simulink model "PMSM_FOC_INVERTER_COMPARISON"  (R2023b)
settings: Solver=VariableStepAuto  StartTime=0.0  StopTime=1  RelTol=1e-3
InitFcn:
  | Ld = 1.7e-3;
  | Lq = 3.2e-3;
  | Rs = 0.02;
  | Lambda_m = 0.2205;
  | J = 0.0027;
  | P = 4;
  | B = 0.001;
  | Vdc = 500;
libraries: slpidlib x9, spsControlledVoltageSourceLib x3, spsGroundLib x3, spsVoltageMeasurementLib x3, spsDCVoltageSourceLib x1, spsPermanentMagnetSynchronousMachineLib x1, spsUniversalBridgeLib x1, sps_lib x1, spsTriangleGeneratorLib x1
(part 2 of 2)

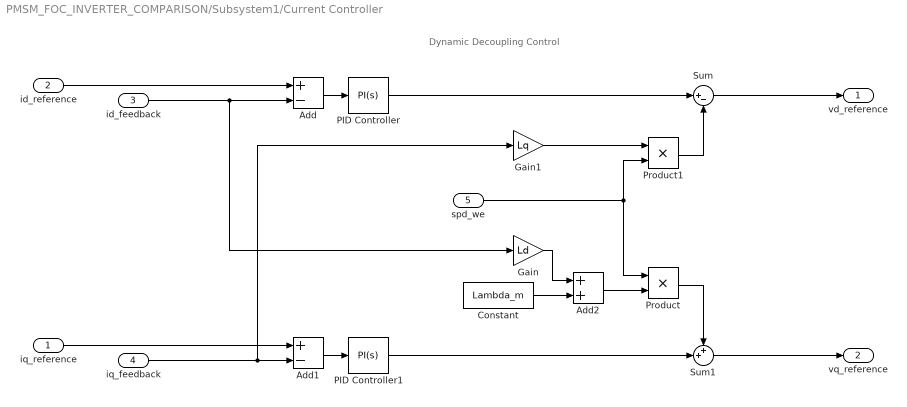
== system PMSM_FOC_INVERTER_COMPARISON/Subsystem1/Current Controller ==
  note: Dynamic Decoupling Control
  iq_reference : Inport  SampleTime=1e-4
  id_reference : Inport  Port=2  SampleTime=1e-4
  id_feedback : Inport  Port=3  SampleTime=1e-4
  iq_feedback : Inport  Port=4  SampleTime=1e-4
  spd_we : Inport  Port=5  SampleTime=1e-4
  Add : Sum  Inputs=+-
  Add1 : Sum  Inputs=+-
  Add2 : Sum
  Constant : Constant  Value=Lambda_m  SampleTime=1e-4
  Gain : Gain  Gain=Ld
  Gain1 : Gain  Gain=Lq
  PID Controller : slpidlib/PID Controller  Controller=PI  Form=Parallel  TimeDomain=Continuous-time  UseExternalTs=off  SampleTime=-1  IntegratorMethod=Forward Euler  FilterMethod=Forward Euler  ControllerParametersSource=internal  P=7.74  I=26.84  UseKiTs=off  D=0  N=100  UseFilter=on  TunerSelectOption=Transfer Function Based (PID Tuner App)  InitialConditionSource=internal  InitialConditionForIntegrator=0  InitialConditionForFilter=0  DifferentiatorICPrevScaledInput=0  ExternalReset=none  TrackingMode=off  Kt=1  LimitOutput=off  SatLimitsSource=internal  UpperSaturationLimit=inf  LowerSaturationLimit=-inf  LinearizeAsGain=on  AntiWindupMode=none  Kb=1  LimitIntegrator=off  UpperIntegratorSaturationLimit=inf  LowerIntegratorSaturationLimit=-inf  POutMin=[]  POutMax=[]  IOutMin=[]  IOutMax=[]  DOutMin=[]  DOutMax=[]  NOutMin=[]  NOutMax=[]  SumOutMin=[]  SumOutMax=[]  SaturationOutMin=[]  SaturationOutMax=[]  PParamMin=[]  PParamMax=[]  IParamMin=[]  IParamMax=[]  DParamMin=[]  DParamMax=[]  NParamMin=[]  NParamMax=[]  KbParamMin=[]  KbParamMax=[]  KtParamMin=[]  KtParamMax=[]  KbOutMin=[]  KbOutMax=[]  KtOutMin=[]  KtOutMax=[]  IntegratorOutMin=[]  IntegratorOutMax=[]  FilterOutMin=[]  FilterOutMax=[]  SumI1OutMin=[]  SumI1OutMax=[]  SumI2OutMin=[]  SumI2OutMax=[]  SumI3OutMin=[]  SumI3OutMax=[]  SumI4OutMin=[]  SumI4OutMax=[]  SumDOutMin=[]  SumDOutMax=[]  DifferentiatorOutMin=[]  DifferentiatorOutMax=[]  FilterDiffOutCoefMin=[]  FilterDiffOutCoefMax=[]  ReciprocalOutMin=[]  ReciprocalOutMax=[]  SumDenOutMin=[]  SumDenOutMax=[]  SumNumOutMin=[]  SumNumOutMax=[]  DivideOutMin=[]  DivideOutMax=[]  UdiffTsProdOutMin=[]  UdiffTsProdOutMax=[]  NTsProdOutMin=[]  NTsProdOutMax=[]  UintegralTsProdOutMin=[]  UintegralTsProdOutMax=[]  UngainTsProdOutMin=[]  UngainTsProdOutMax=[]  ClampingZeroOutDataTypeStr=Inherit: Inherit via back propagation  ClampingZeroOutMin=[]  ClampingZeroOutMax=[]  FilterDenConstantOutDataTypeStr=Inherit: Inherit via back propagation  FilterDenConstantOutMin=[]  FilterDenConstantOutMax=[]  PCopyOutDataTypeStr=Inherit: Inherit via back propagation  PCopyOutMin=[]  PCopyOutMax=[]  NCopyOutDataTypeStr=Inherit: Inherit via back propagation  NCopyOutMin=[]  NCopyOutMax=[]  IntegratorContinuousStateAttributes=''  IntegratorStateMustResolveToSignalObject=off  IntegratorRTWStateStorageClass=Auto  FilterContinuousStateAttributes=''  FilterStateMustResolveToSignalObject=off  FilterRTWStateStorageClass=Auto  ParallelPVariant=InternalParameters  IdealPVariant=Disabled  IVariant=InternalParameters  DVariant=Disabled  IntegratorVariant=Continuous  SatVariant=Disabled  AWVariant=Passthrough  PCopyVariant=Disabled  TRVariant=Disabled  FdbkBlocksVariant=Forward  IdealPFdbkVariant=Disabled  SatFdbkVariant=Disabled  DerivativeFilterVariant=Disabled  NVariant=Disabled  NCopyVariant=Disabled_SignalSpec  FilterICVariant=Disabled  IntegratorICVariant=InternalICs  ExternalResetVariant=Disabled  TRSumVariant=Passthrough  SumFdbkVariant=Disabled  SumVariant=Sum_PI  TsampFilterVariant=InternalTs  TsampNgainVariant=Passthrough  TsampIntegralVariant=Disabled_SignalSpec  ExternalSaturationOutDataTypeStr=Inherit: Same as second input
  PID Controller1 : slpidlib/PID Controller  Controller=PI  Form=Parallel  TimeDomain=Continuous-time  UseExternalTs=off  SampleTime=-1  IntegratorMethod=Forward Euler  FilterMethod=Forward Euler  ControllerParametersSource=internal  P=7.74  I=26.84  UseKiTs=off  D=0  N=100  UseFilter=on  TunerSelectOption=Transfer Function Based (PID Tuner App)  InitialConditionSource=internal  InitialConditionForIntegrator=0  InitialConditionForFilter=0  DifferentiatorICPrevScaledInput=0  ExternalReset=none  TrackingMode=off  Kt=1  LimitOutput=off  SatLimitsSource=internal  UpperSaturationLimit=inf  LowerSaturationLimit=-inf  LinearizeAsGain=on  AntiWindupMode=none  Kb=1  LimitIntegrator=off  UpperIntegratorSaturationLimit=inf  LowerIntegratorSaturationLimit=-inf  POutMin=[]  POutMax=[]  IOutMin=[]  IOutMax=[]  DOutMin=[]  DOutMax=[]  NOutMin=[]  NOutMax=[]  SumOutMin=[]  SumOutMax=[]  SaturationOutMin=[]  SaturationOutMax=[]  PParamMin=[]  PParamMax=[]  IParamMin=[]  IParamMax=[]  DParamMin=[]  DParamMax=[]  NParamMin=[]  NParamMax=[]  KbParamMin=[]  KbParamMax=[]  KtParamMin=[]  KtParamMax=[]  KbOutMin=[]  KbOutMax=[]  KtOutMin=[]  KtOutMax=[]  IntegratorOutMin=[]  IntegratorOutMax=[]  FilterOutMin=[]  FilterOutMax=[]  SumI1OutMin=[]  SumI1OutMax=[]  SumI2OutMin=[]  SumI2OutMax=[]  SumI3OutMin=[]  SumI3OutMax=[]  SumI4OutMin=[]  SumI4OutMax=[]  SumDOutMin=[]  SumDOutMax=[]  DifferentiatorOutMin=[]  DifferentiatorOutMax=[]  FilterDiffOutCoefMin=[]  FilterDiffOutCoefMax=[]  ReciprocalOutMin=[]  ReciprocalOutMax=[]  SumDenOutMin=[]  SumDenOutMax=[]  SumNumOutMin=[]  SumNumOutMax=[]  DivideOutMin=[]  DivideOutMax=[]  UdiffTsProdOutMin=[]  UdiffTsProdOutMax=[]  NTsProdOutMin=[]  NTsProdOutMax=[]  UintegralTsProdOutMin=[]  UintegralTsProdOutMax=[]  UngainTsProdOutMin=[]  UngainTsProdOutMax=[]  ClampingZeroOutDataTypeStr=Inherit: Inherit via back propagation  ClampingZeroOutMin=[]  ClampingZeroOutMax=[]  FilterDenConstantOutDataTypeStr=Inherit: Inherit via back propagation  FilterDenConstantOutMin=[]  FilterDenConstantOutMax=[]  PCopyOutDataTypeStr=Inherit: Inherit via back propagation  PCopyOutMin=[]  PCopyOutMax=[]  NCopyOutDataTypeStr=Inherit: Inherit via back propagation  NCopyOutMin=[]  NCopyOutMax=[]  IntegratorContinuousStateAttributes=''  IntegratorStateMustResolveToSignalObject=off  IntegratorRTWStateStorageClass=Auto  FilterContinuousStateAttributes=''  FilterStateMustResolveToSignalObject=off  FilterRTWStateStorageClass=Auto  ParallelPVariant=InternalParameters  IdealPVariant=Disabled  IVariant=InternalParameters  DVariant=Disabled  IntegratorVariant=Continuous  SatVariant=Disabled  AWVariant=Passthrough  PCopyVariant=Disabled  TRVariant=Disabled  FdbkBlocksVariant=Forward  IdealPFdbkVariant=Disabled  SatFdbkVariant=Disabled  DerivativeFilterVariant=Disabled  NVariant=Disabled  NCopyVariant=Disabled_SignalSpec  FilterICVariant=Disabled  IntegratorICVariant=InternalICs  ExternalResetVariant=Disabled  TRSumVariant=Passthrough  SumFdbkVariant=Disabled  SumVariant=Sum_PI  TsampFilterVariant=InternalTs  TsampNgainVariant=Passthrough  TsampIntegralVariant=Disabled_SignalSpec  ExternalSaturationOutDataTypeStr=Inherit: Same as second input
  Product : Product
  Product1 : Product
  Sum : Sum  Inputs=|+-
  Sum1 : Sum  Inputs=++|
  vd_reference : Outport  SampleTime=1e-4  VectorParamsAs1DForOutWhenUnconnected=off
  vq_reference : Outport  Port=2  SampleTime=1e-4  VectorParamsAs1DForOutWhenUnconnected=off
  wires:
  Product/1 -> Sum1/1
  Product1/1 -> Sum/2
  Gain1/1 -> Product1/1
  spd_we/1 -> Product/1, Product1/2
  Add2/1 -> Product/2
  Constant/1 -> Add2/2
  Gain/1 -> Add2/1
  PID Controller1/1 -> Sum1/2
  Sum1/1 -> vq_reference/1
  iq_reference/1 -> Add1/1
  Add1/1 -> PID Controller1/1
  id_reference/1 -> Add/1
  iq_feedback/1 -> Add1/2, Gain1/1
  Add/1 -> PID Controller/1
  id_feedback/1 -> Add/2, Gain/1
  PID Controller/1 -> Sum/1
  Sum/1 -> vd_reference/1

== system PMSM_FOC_INVERTER_COMPARISON/Subsystem1/Subsystem ==
  Speed_CMD : Inport
  Speed_feedback : Inport  Port=2
  Gain : Gain  Gain=2/(3*P*Lambda_m)
  Id_CMD : Constant  Value=0
  PID Controller1 : slpidlib/PID Controller  Controller=PI  Form=Parallel  TimeDomain=Continuous-time  UseExternalTs=off  SampleTime=-1  IntegratorMethod=Forward Euler  FilterMethod=Forward Euler  ControllerParametersSource=internal  P=0.1  I=0.1  UseKiTs=off  D=0  N=100  UseFilter=on  TunerSelectOption=Transfer Function Based (PID Tuner App)  InitialConditionSource=internal  InitialConditionForIntegrator=0  InitialConditionForFilter=0  DifferentiatorICPrevScaledInput=0  ExternalReset=none  TrackingMode=off  Kt=1  LimitOutput=off  SatLimitsSource=internal  UpperSaturationLimit=inf  LowerSaturationLimit=-inf  LinearizeAsGain=on  AntiWindupMode=none  Kb=1  LimitIntegrator=off  UpperIntegratorSaturationLimit=inf  LowerIntegratorSaturationLimit=-inf  POutMin=[]  POutMax=[]  IOutMin=[]  IOutMax=[]  DOutMin=[]  DOutMax=[]  NOutMin=[]  NOutMax=[]  SumOutMin=[]  SumOutMax=[]  SaturationOutMin=[]  SaturationOutMax=[]  PParamMin=[]  PParamMax=[]  IParamMin=[]  IParamMax=[]  DParamMin=[]  DParamMax=[]  NParamMin=[]  NParamMax=[]  KbParamMin=[]  KbParamMax=[]  KtParamMin=[]  KtParamMax=[]  KbOutMin=[]  KbOutMax=[]  KtOutMin=[]  KtOutMax=[]  IntegratorOutMin=[]  IntegratorOutMax=[]  FilterOutMin=[]  FilterOutMax=[]  SumI1OutMin=[]  SumI1OutMax=[]  SumI2OutMin=[]  SumI2OutMax=[]  SumI3OutMin=[]  SumI3OutMax=[]  SumI4OutMin=[]  SumI4OutMax=[]  SumDOutMin=[]  SumDOutMax=[]  DifferentiatorOutMin=[]  DifferentiatorOutMax=[]  FilterDiffOutCoefMin=[]  FilterDiffOutCoefMax=[]  ReciprocalOutMin=[]  ReciprocalOutMax=[]  SumDenOutMin=[]  SumDenOutMax=[]  SumNumOutMin=[]  SumNumOutMax=[]  DivideOutMin=[]  DivideOutMax=[]  UdiffTsProdOutMin=[]  UdiffTsProdOutMax=[]  NTsProdOutMin=[]  NTsProdOutMax=[]  UintegralTsProdOutMin=[]  UintegralTsProdOutMax=[]  UngainTsProdOutMin=[]  UngainTsProdOutMax=[]  ClampingZeroOutDataTypeStr=Inherit: Inherit via back propagation  ClampingZeroOutMin=[]  ClampingZeroOutMax=[]  FilterDenConstantOutDataTypeStr=Inherit: Inherit via back propagation  FilterDenConstantOutMin=[]  FilterDenConstantOutMax=[]  PCopyOutDataTypeStr=Inherit: Inherit via back propagation  PCopyOutMin=[]  PCopyOutMax=[]  NCopyOutDataTypeStr=Inherit: Inherit via back propagation  NCopyOutMin=[]  NCopyOutMax=[]  IntegratorContinuousStateAttributes=''  IntegratorStateMustResolveToSignalObject=off  IntegratorRTWStateStorageClass=Auto  FilterContinuousStateAttributes=''  FilterStateMustResolveToSignalObject=off  FilterRTWStateStorageClass=Auto  ParallelPVariant=InternalParameters  IdealPVariant=Disabled  IVariant=InternalParameters  DVariant=Disabled  IntegratorVariant=Continuous  SatVariant=Disabled  AWVariant=Passthrough  PCopyVariant=Disabled  TRVariant=Disabled  FdbkBlocksVariant=Forward  IdealPFdbkVariant=Disabled  SatFdbkVariant=Disabled  DerivativeFilterVariant=Disabled  NVariant=Disabled  NCopyVariant=Disabled_SignalSpec  FilterICVariant=Disabled  IntegratorICVariant=InternalICs  ExternalResetVariant=Disabled  TRSumVariant=Passthrough  SumFdbkVariant=Disabled  SumVariant=Sum_PI  TsampFilterVariant=InternalTs  TsampNgainVariant=Passthrough  TsampIntegralVariant=Disabled_SignalSpec  ExternalSaturationOutDataTypeStr=Inherit: Same as second input
  Sum : Sum  Inputs=|+-
  Iq_ref : Outport
  Id_ref : Outport  Port=2
  wires:
  Gain/1 -> Iq_ref/1
  PID Controller1/1 -> Gain/1
  Id_CMD/1 -> Id_ref/1
  Speed_CMD/1 -> Sum/1
  Sum/1 -> PID Controller1/1
  Speed_feedback/1 -> Sum/2

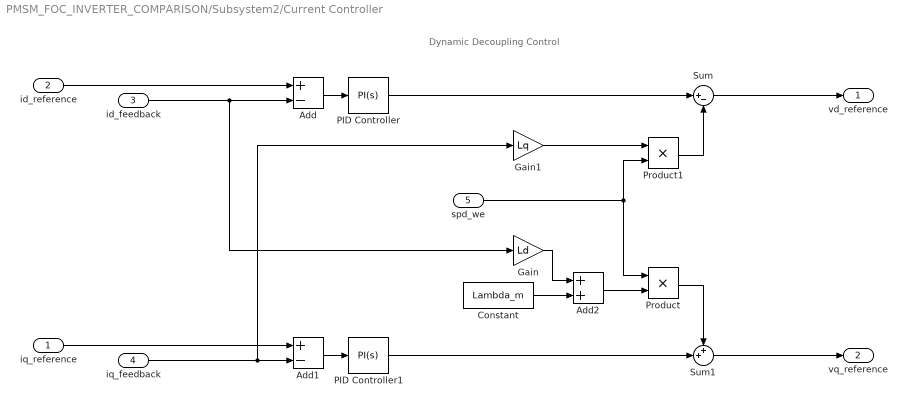
== system PMSM_FOC_INVERTER_COMPARISON/Subsystem2/Current Controller ==
  note: Dynamic Decoupling Control
  iq_reference : Inport  SampleTime=1e-4
  id_reference : Inport  Port=2  SampleTime=1e-4
  id_feedback : Inport  Port=3  SampleTime=1e-4
  iq_feedback : Inport  Port=4  SampleTime=1e-4
  spd_we : Inport  Port=5  SampleTime=1e-4
  Add : Sum  Inputs=+-
  Add1 : Sum  Inputs=+-
  Add2 : Sum
  Constant : Constant  Value=Lambda_m  SampleTime=1e-4
  Gain : Gain  Gain=Ld
  Gain1 : Gain  Gain=Lq
  PID Controller : slpidlib/PID Controller  Controller=PI  Form=Parallel  TimeDomain=Continuous-time  UseExternalTs=off  SampleTime=-1  IntegratorMethod=Forward Euler  FilterMethod=Forward Euler  ControllerParametersSource=internal  P=7.74  I=26.84  UseKiTs=off  D=0  N=100  UseFilter=on  TunerSelectOption=Transfer Function Based (PID Tuner App)  InitialConditionSource=internal  InitialConditionForIntegrator=0  InitialConditionForFilter=0  DifferentiatorICPrevScaledInput=0  ExternalReset=none  TrackingMode=off  Kt=1  LimitOutput=off  SatLimitsSource=internal  UpperSaturationLimit=inf  LowerSaturationLimit=-inf  LinearizeAsGain=on  AntiWindupMode=none  Kb=1  LimitIntegrator=off  UpperIntegratorSaturationLimit=inf  LowerIntegratorSaturationLimit=-inf  POutMin=[]  POutMax=[]  IOutMin=[]  IOutMax=[]  DOutMin=[]  DOutMax=[]  NOutMin=[]  NOutMax=[]  SumOutMin=[]  SumOutMax=[]  SaturationOutMin=[]  SaturationOutMax=[]  PParamMin=[]  PParamMax=[]  IParamMin=[]  IParamMax=[]  DParamMin=[]  DParamMax=[]  NParamMin=[]  NParamMax=[]  KbParamMin=[]  KbParamMax=[]  KtParamMin=[]  KtParamMax=[]  KbOutMin=[]  KbOutMax=[]  KtOutMin=[]  KtOutMax=[]  IntegratorOutMin=[]  IntegratorOutMax=[]  FilterOutMin=[]  FilterOutMax=[]  SumI1OutMin=[]  SumI1OutMax=[]  SumI2OutMin=[]  SumI2OutMax=[]  SumI3OutMin=[]  SumI3OutMax=[]  SumI4OutMin=[]  SumI4OutMax=[]  SumDOutMin=[]  SumDOutMax=[]  DifferentiatorOutMin=[]  DifferentiatorOutMax=[]  FilterDiffOutCoefMin=[]  FilterDiffOutCoefMax=[]  ReciprocalOutMin=[]  ReciprocalOutMax=[]  SumDenOutMin=[]  SumDenOutMax=[]  SumNumOutMin=[]  SumNumOutMax=[]  DivideOutMin=[]  DivideOutMax=[]  UdiffTsProdOutMin=[]  UdiffTsProdOutMax=[]  NTsProdOutMin=[]  NTsProdOutMax=[]  UintegralTsProdOutMin=[]  UintegralTsProdOutMax=[]  UngainTsProdOutMin=[]  UngainTsProdOutMax=[]  ClampingZeroOutDataTypeStr=Inherit: Inherit via back propagation  ClampingZeroOutMin=[]  ClampingZeroOutMax=[]  FilterDenConstantOutDataTypeStr=Inherit: Inherit via back propagation  FilterDenConstantOutMin=[]  FilterDenConstantOutMax=[]  PCopyOutDataTypeStr=Inherit: Inherit via back propagation  PCopyOutMin=[]  PCopyOutMax=[]  NCopyOutDataTypeStr=Inherit: Inherit via back propagation  NCopyOutMin=[]  NCopyOutMax=[]  IntegratorContinuousStateAttributes=''  IntegratorStateMustResolveToSignalObject=off  IntegratorRTWStateStorageClass=Auto  FilterContinuousStateAttributes=''  FilterStateMustResolveToSignalObject=off  FilterRTWStateStorageClass=Auto  ParallelPVariant=InternalParameters  IdealPVariant=Disabled  IVariant=InternalParameters  DVariant=Disabled  IntegratorVariant=Continuous  SatVariant=Disabled  AWVariant=Passthrough  PCopyVariant=Disabled  TRVariant=Disabled  FdbkBlocksVariant=Forward  IdealPFdbkVariant=Disabled  SatFdbkVariant=Disabled  DerivativeFilterVariant=Disabled  NVariant=Disabled  NCopyVariant=Disabled_SignalSpec  FilterICVariant=Disabled  IntegratorICVariant=InternalICs  ExternalResetVariant=Disabled  TRSumVariant=Passthrough  SumFdbkVariant=Disabled  SumVariant=Sum_PI  TsampFilterVariant=InternalTs  TsampNgainVariant=Passthrough  TsampIntegralVariant=Disabled_SignalSpec  ExternalSaturationOutDataTypeStr=Inherit: Same as second input
  PID Controller1 : slpidlib/PID Controller  Controller=PI  Form=Parallel  TimeDomain=Continuous-time  UseExternalTs=off  SampleTime=-1  IntegratorMethod=Forward Euler  FilterMethod=Forward Euler  ControllerParametersSource=internal  P=7.74  I=26.84  UseKiTs=off  D=0  N=100  UseFilter=on  TunerSelectOption=Transfer Function Based (PID Tuner App)  InitialConditionSource=internal  InitialConditionForIntegrator=0  InitialConditionForFilter=0  DifferentiatorICPrevScaledInput=0  ExternalReset=none  TrackingMode=off  Kt=1  LimitOutput=off  SatLimitsSource=internal  UpperSaturationLimit=inf  LowerSaturationLimit=-inf  LinearizeAsGain=on  AntiWindupMode=none  Kb=1  LimitIntegrator=off  UpperIntegratorSaturationLimit=inf  LowerIntegratorSaturationLimit=-inf  POutMin=[]  POutMax=[]  IOutMin=[]  IOutMax=[]  DOutMin=[]  DOutMax=[]  NOutMin=[]  NOutMax=[]  SumOutMin=[]  SumOutMax=[]  SaturationOutMin=[]  SaturationOutMax=[]  PParamMin=[]  PParamMax=[]  IParamMin=[]  IParamMax=[]  DParamMin=[]  DParamMax=[]  NParamMin=[]  NParamMax=[]  KbParamMin=[]  KbParamMax=[]  KtParamMin=[]  KtParamMax=[]  KbOutMin=[]  KbOutMax=[]  KtOutMin=[]  KtOutMax=[]  IntegratorOutMin=[]  IntegratorOutMax=[]  FilterOutMin=[]  FilterOutMax=[]  SumI1OutMin=[]  SumI1OutMax=[]  SumI2OutMin=[]  SumI2OutMax=[]  SumI3OutMin=[]  SumI3OutMax=[]  SumI4OutMin=[]  SumI4OutMax=[]  SumDOutMin=[]  SumDOutMax=[]  DifferentiatorOutMin=[]  DifferentiatorOutMax=[]  FilterDiffOutCoefMin=[]  FilterDiffOutCoefMax=[]  ReciprocalOutMin=[]  ReciprocalOutMax=[]  SumDenOutMin=[]  SumDenOutMax=[]  SumNumOutMin=[]  SumNumOutMax=[]  DivideOutMin=[]  DivideOutMax=[]  UdiffTsProdOutMin=[]  UdiffTsProdOutMax=[]  NTsProdOutMin=[]  NTsProdOutMax=[]  UintegralTsProdOutMin=[]  UintegralTsProdOutMax=[]  UngainTsProdOutMin=[]  UngainTsProdOutMax=[]  ClampingZeroOutDataTypeStr=Inherit: Inherit via back propagation  ClampingZeroOutMin=[]  ClampingZeroOutMax=[]  FilterDenConstantOutDataTypeStr=Inherit: Inherit via back propagation  FilterDenConstantOutMin=[]  FilterDenConstantOutMax=[]  PCopyOutDataTypeStr=Inherit: Inherit via back propagation  PCopyOutMin=[]  PCopyOutMax=[]  NCopyOutDataTypeStr=Inherit: Inherit via back propagation  NCopyOutMin=[]  NCopyOutMax=[]  IntegratorContinuousStateAttributes=''  IntegratorStateMustResolveToSignalObject=off  IntegratorRTWStateStorageClass=Auto  FilterContinuousStateAttributes=''  FilterStateMustResolveToSignalObject=off  FilterRTWStateStorageClass=Auto  ParallelPVariant=InternalParameters  IdealPVariant=Disabled  IVariant=InternalParameters  DVariant=Disabled  IntegratorVariant=Continuous  SatVariant=Disabled  AWVariant=Passthrough  PCopyVariant=Disabled  TRVariant=Disabled  FdbkBlocksVariant=Forward  IdealPFdbkVariant=Disabled  SatFdbkVariant=Disabled  DerivativeFilterVariant=Disabled  NVariant=Disabled  NCopyVariant=Disabled_SignalSpec  FilterICVariant=Disabled  IntegratorICVariant=InternalICs  ExternalResetVariant=Disabled  TRSumVariant=Passthrough  SumFdbkVariant=Disabled  SumVariant=Sum_PI  TsampFilterVariant=InternalTs  TsampNgainVariant=Passthrough  TsampIntegralVariant=Disabled_SignalSpec  ExternalSaturationOutDataTypeStr=Inherit: Same as second input
  Product : Product
  Product1 : Product
  Sum : Sum  Inputs=|+-
  Sum1 : Sum  Inputs=++|
  vd_reference : Outport  SampleTime=1e-4  VectorParamsAs1DForOutWhenUnconnected=off
  vq_reference : Outport  Port=2  SampleTime=1e-4  VectorParamsAs1DForOutWhenUnconnected=off
  wires:
  Sum/1 -> vd_reference/1
  PID Controller/1 -> Sum/1
  id_feedback/1 -> Gain/1, Add/2
  Add/1 -> PID Controller/1
  iq_feedback/1 -> Gain1/1, Add1/2
  id_reference/1 -> Add/1
  Add1/1 -> PID Controller1/1
  iq_reference/1 -> Add1/1
  Sum1/1 -> vq_reference/1
  PID Controller1/1 -> Sum1/2
  Gain/1 -> Add2/1
  Constant/1 -> Add2/2
  Add2/1 -> Product/2
  spd_we/1 -> Product1/2, Product/1
  Gain1/1 -> Product1/1
  Product1/1 -> Sum/2
  Product/1 -> Sum1/1

== system PMSM_FOC_INVERTER_COMPARISON/Subsystem2/Subsystem ==
  Speed_CMD : Inport
  Speed_feedback : Inport  Port=2
  Gain : Gain  Gain=2/(3*P*Lambda_m)
  Id_CMD : Constant  Value=0
  PID Controller1 : slpidlib/PID Controller  Controller=PI  Form=Parallel  TimeDomain=Continuous-time  UseExternalTs=off  SampleTime=-1  IntegratorMethod=Forward Euler  FilterMethod=Forward Euler  ControllerParametersSource=internal  P=0.1  I=0.1  UseKiTs=off  D=0  N=100  UseFilter=on  TunerSelectOption=Transfer Function Based (PID Tuner App)  InitialConditionSource=internal  InitialConditionForIntegrator=0  InitialConditionForFilter=0  DifferentiatorICPrevScaledInput=0  ExternalReset=none  TrackingMode=off  Kt=1  LimitOutput=off  SatLimitsSource=internal  UpperSaturationLimit=inf  LowerSaturationLimit=-inf  LinearizeAsGain=on  AntiWindupMode=none  Kb=1  LimitIntegrator=off  UpperIntegratorSaturationLimit=inf  LowerIntegratorSaturationLimit=-inf  POutMin=[]  POutMax=[]  IOutMin=[]  IOutMax=[]  DOutMin=[]  DOutMax=[]  NOutMin=[]  NOutMax=[]  SumOutMin=[]  SumOutMax=[]  SaturationOutMin=[]  SaturationOutMax=[]  PParamMin=[]  PParamMax=[]  IParamMin=[]  IParamMax=[]  DParamMin=[]  DParamMax=[]  NParamMin=[]  NParamMax=[]  KbParamMin=[]  KbParamMax=[]  KtParamMin=[]  KtParamMax=[]  KbOutMin=[]  KbOutMax=[]  KtOutMin=[]  KtOutMax=[]  IntegratorOutMin=[]  IntegratorOutMax=[]  FilterOutMin=[]  FilterOutMax=[]  SumI1OutMin=[]  SumI1OutMax=[]  SumI2OutMin=[]  SumI2OutMax=[]  SumI3OutMin=[]  SumI3OutMax=[]  SumI4OutMin=[]  SumI4OutMax=[]  SumDOutMin=[]  SumDOutMax=[]  DifferentiatorOutMin=[]  DifferentiatorOutMax=[]  FilterDiffOutCoefMin=[]  FilterDiffOutCoefMax=[]  ReciprocalOutMin=[]  ReciprocalOutMax=[]  SumDenOutMin=[]  SumDenOutMax=[]  SumNumOutMin=[]  SumNumOutMax=[]  DivideOutMin=[]  DivideOutMax=[]  UdiffTsProdOutMin=[]  UdiffTsProdOutMax=[]  NTsProdOutMin=[]  NTsProdOutMax=[]  UintegralTsProdOutMin=[]  UintegralTsProdOutMax=[]  UngainTsProdOutMin=[]  UngainTsProdOutMax=[]  ClampingZeroOutDataTypeStr=Inherit: Inherit via back propagation  ClampingZeroOutMin=[]  ClampingZeroOutMax=[]  FilterDenConstantOutDataTypeStr=Inherit: Inherit via back propagation  FilterDenConstantOutMin=[]  FilterDenConstantOutMax=[]  PCopyOutDataTypeStr=Inherit: Inherit via back propagation  PCopyOutMin=[]  PCopyOutMax=[]  NCopyOutDataTypeStr=Inherit: Inherit via back propagation  NCopyOutMin=[]  NCopyOutMax=[]  IntegratorContinuousStateAttributes=''  IntegratorStateMustResolveToSignalObject=off  IntegratorRTWStateStorageClass=Auto  FilterContinuousStateAttributes=''  FilterStateMustResolveToSignalObject=off  FilterRTWStateStorageClass=Auto  ParallelPVariant=InternalParameters  IdealPVariant=Disabled  IVariant=InternalParameters  DVariant=Disabled  IntegratorVariant=Continuous  SatVariant=Disabled  AWVariant=Passthrough  PCopyVariant=Disabled  TRVariant=Disabled  FdbkBlocksVariant=Forward  IdealPFdbkVariant=Disabled  SatFdbkVariant=Disabled  DerivativeFilterVariant=Disabled  NVariant=Disabled  NCopyVariant=Disabled_SignalSpec  FilterICVariant=Disabled  IntegratorICVariant=InternalICs  ExternalResetVariant=Disabled  TRSumVariant=Passthrough  SumFdbkVariant=Disabled  SumVariant=Sum_PI  TsampFilterVariant=InternalTs  TsampNgainVariant=Passthrough  TsampIntegralVariant=Disabled_SignalSpec  ExternalSaturationOutDataTypeStr=Inherit: Same as second input
  Sum : Sum  Inputs=|+-
  Iq_ref : Outport
  Id_ref : Outport  Port=2
  wires:
  Speed_feedback/1 -> Sum/2
  Sum/1 -> PID Controller1/1
  Speed_CMD/1 -> Sum/1
  Id_CMD/1 -> Id_ref/1
  PID Controller1/1 -> Gain/1
  Gain/1 -> Iq_ref/1

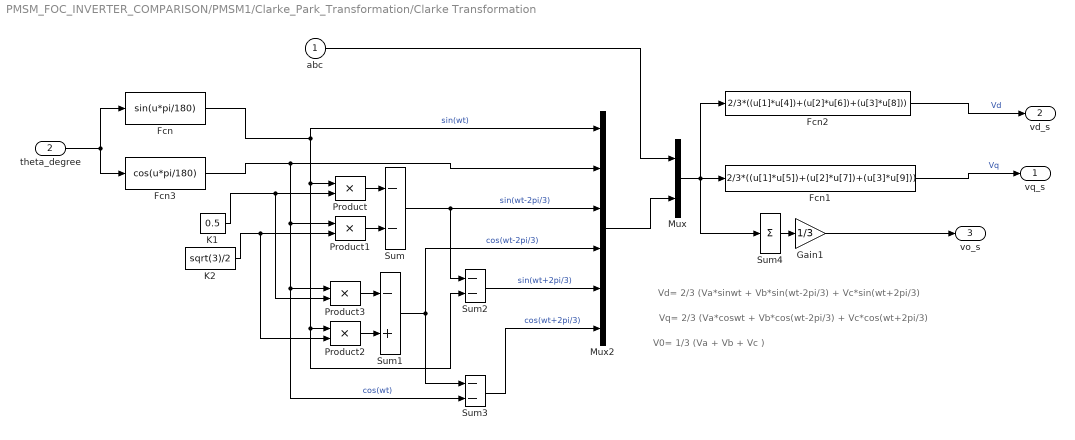
== system PMSM_FOC_INVERTER_COMPARISON/PMSM1/Clarke_Park_Transformation/Clarke Transformation ==
  note: Vq= 2/3 (Va*coswt + Vb*cos(wt-2pi/3) + Vc*cos(wt+2pi/3)
  note: V0= 1/3 (Va + Vb + Vc )
  note: Vd= 2/3 (Va*sinwt + Vb*sin(wt-2pi/3) + Vc*sin(wt+2pi/3)
  abc : Inport  PortDimensions=3
  theta_degree : Inport  Port=2
  Fcn : Fcn  Expr=sin(u*pi/180)
  Fcn1 : Fcn  Expr=2/3*((u[1]*u[5])+(u[2]*u[7])+(u[3]*u[9]))
  Fcn2 : Fcn  Expr=2/3*((u[1]*u[4])+(u[2]*u[6])+(u[3]*u[8]))
  Fcn3 : Fcn  Expr=cos(u*pi/180)
  Gain1 : Gain  Gain=1/3  SaturateOnIntegerOverflow=on  OutDataTypeStr=Inherit: Same as input  ParamDataTypeStr=Inherit: Same as input
  K1 : Constant  Value=0.5
  K2 : Constant  Value=sqrt(3)/2
  Mux : Mux  Inputs=2
  Mux2 : Mux  Inputs=6
  Product{,1..3} (4 alike) : Product  InputSameDT=on  SaturateOnIntegerOverflow=on  OutDataTypeStr=Inherit: Same as first input
  Sum : Sum  Inputs=--  InputSameDT=on  SaturateOnIntegerOverflow=on  OutDataTypeStr=Inherit: Same as first input
  Sum1 : Sum  Inputs=-+  InputSameDT=on  SaturateOnIntegerOverflow=on  OutDataTypeStr=Inherit: Same as first input
  Sum2 : Sum  Inputs=--  InputSameDT=on  SaturateOnIntegerOverflow=on  OutDataTypeStr=Inherit: Same as first input
  Sum3 : Sum  Inputs=--  InputSameDT=on  SaturateOnIntegerOverflow=on  OutDataTypeStr=Inherit: Same as first input
  Sum4 : Sum  Inputs=1  InputSameDT=on  SaturateOnIntegerOverflow=on  OutDataTypeStr=Inherit: Same as first input
  vq_s : Outport
  vd_s : Outport  Port=2
  vo_s : Outport  Port=3
  wires:
  Gain1/1 -> vo_s/1
  Mux/1 -> Sum4/1, Fcn1/1, Fcn2/1
  theta_degree/1 -> Fcn/1, Fcn3/1
  Sum3/1 -> Mux2/6  "cos(wt+2pi/3)"
  Fcn2/1 -> vd_s/1  "Vd"
  Product3/1 -> Sum1/1
  Sum4/1 -> Gain1/1
  abc/1 -> Mux/1
  Product/1 -> Sum/1
  Mux2/1 -> Mux/2
  Product2/1 -> Sum1/2
  Product1/1 -> Sum/2
  K1/1 -> Product3/2, Product/2
  Sum1/1 -> Sum3/1, Mux2/4  "cos(wt-2pi/3)"
  Fcn/1 -> Mux2/1, Sum2/2, Product2/1, Product/1  "sin(wt)"
  Sum2/1 -> Mux2/5  "sin(wt+2pi/3)"
  K2/1 -> Product2/2, Product1/2
  Fcn3/1 -> Mux2/2, Product1/1, Product3/1, Sum3/2  "cos(wt)"
  Fcn1/1 -> vq_s/1  "Vq"
  Sum/1 -> Sum2/1, Mux2/3  "sin(wt-2pi/3)"

== system PMSM_FOC_INVERTER_COMPARISON/PMSM1/Clarke_Park_Transformation/Park Transformation ==
  qs_s : Inport
  ds_s : Inport  Port=2
  cos theta_e : Inport  Port=3
  Sin theta_e : Inport  Port=4
  Add : Sum  Inputs=+-
  Add1 : Sum
  Product{,1..3} (4 alike) : Product  RndMeth=Zero
  qs_r : Outport
  ds_r : Outport  Port=2
  wires:
  Product2/1 -> Add1/2
  Product3/1 -> Add1/1
  Add/1 -> qs_r/1
  qs_s/1 -> Product3/1, Product/1
  Product/1 -> Add/1
  Add1/1 -> ds_r/1
  ds_s/1 -> Product2/1, Product1/1
  Product1/1 -> Add/2
  Sin theta_e/1 -> Product3/2, Product1/2
  cos theta_e/1 -> Product2/2, Product/2

== system PMSM_FOC_INVERTER_COMPARISON/PMSM1/Clarke_Park_Transformation/Subsystem ==
  theta_e : Inport
  Fcn : Fcn  Expr=sin(u)
  Fcn1 : Fcn  Expr=cos(u)
  cos : Outport
  sin : Outport  Port=2
  wires:
  Fcn/1 -> sin/1
  Fcn1/1 -> cos/1
  theta_e/1 -> Fcn1/1, Fcn/1

== system PMSM_FOC_INVERTER_COMPARISON/PMSM1/PMSM Dynamic Model/Electromagnetic Torque ==
  iq : Inport
  id : Inport  Port=2
  Add : Sum
  Gain : Gain  Gain=Ld-Lq
  Gain1 : Gain  Gain=(3/2)*P
  Gain2 : Gain  Gain=Lambda_m
  Product : Product
  Te : Outport
  wires:
  id/1 -> Product/2
  Gain1/1 -> Te/1
  Gain/1 -> Add/1
  iq/1 -> Product/1, Gain2/1
  Product/1 -> Gain/1
  Gain2/1 -> Add/2
  Add/1 -> Gain1/1

== system PMSM_FOC_INVERTER_COMPARISON/PMSM1/PMSM Dynamic Model/Subsystem ==
  Te : Inport
  TL : Inport  Port=2
  Gain : Gain  Gain=1/P
  Integrator : Integrator
  Mechanical_speed_calculations : Subsystem
  Omega_m : Outport
  Theta_m : Outport  Port=2
  Omega_e : Outport  Port=3
  Theta_e : Outport  Port=4
  wires:
  Gain/1 -> Omega_m/1, Integrator/1
  Mechanical_speed_calculations/2(Theta_e) -> Theta_e/1
  Te/1 -> Mechanical_speed_calculations/1(Te)
  Mechanical_speed_calculations/1(Omega_e) -> Omega_e/1, Gain/1
  Integrator/1 -> Theta_m/1
  TL/1 -> Mechanical_speed_calculations/2(TL)

== system PMSM_FOC_INVERTER_COMPARISON/PMSM1/PMSM Dynamic Model/iqd_calculations ==
  vq : Inport
  Omega_e : Inport  Port=2
  vd : Inport  Port=3
  id_calculations : Subsystem
  iq_calculations : Subsystem
  iq : Outport
  id : Outport  Port=2
  wires:
  vd/1 -> id_calculations/1(vd)
  iq_calculations/1(iq) -> id_calculations/3(iq), iq/1
  Omega_e/1 -> id_calculations/2(Omega_e), iq_calculations/2(Omega_e)
  id_calculations/1(id) -> iq_calculations/3(id), id/1
  vq/1 -> iq_calculations/1(vq)

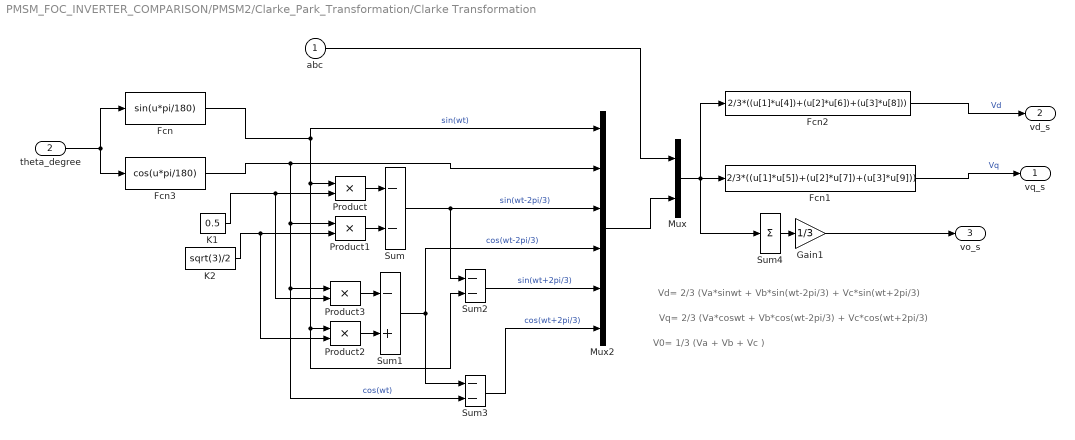
== system PMSM_FOC_INVERTER_COMPARISON/PMSM2/Clarke_Park_Transformation/Clarke Transformation ==
  note: Vd= 2/3 (Va*sinwt + Vb*sin(wt-2pi/3) + Vc*sin(wt+2pi/3)
  note: V0= 1/3 (Va + Vb + Vc )
  note: Vq= 2/3 (Va*coswt + Vb*cos(wt-2pi/3) + Vc*cos(wt+2pi/3)
  abc : Inport  PortDimensions=3
  theta_degree : Inport  Port=2
  Fcn : Fcn  Expr=sin(u*pi/180)
  Fcn1 : Fcn  Expr=2/3*((u[1]*u[5])+(u[2]*u[7])+(u[3]*u[9]))
  Fcn2 : Fcn  Expr=2/3*((u[1]*u[4])+(u[2]*u[6])+(u[3]*u[8]))
  Fcn3 : Fcn  Expr=cos(u*pi/180)
  Gain1 : Gain  Gain=1/3  SaturateOnIntegerOverflow=on  OutDataTypeStr=Inherit: Same as input  ParamDataTypeStr=Inherit: Same as input
  K1 : Constant  Value=0.5
  K2 : Constant  Value=sqrt(3)/2
  Mux : Mux  Inputs=2
  Mux2 : Mux  Inputs=6
  Product{,1..3} (4 alike) : Product  InputSameDT=on  SaturateOnIntegerOverflow=on  OutDataTypeStr=Inherit: Same as first input
  Sum : Sum  Inputs=--  InputSameDT=on  SaturateOnIntegerOverflow=on  OutDataTypeStr=Inherit: Same as first input
  Sum1 : Sum  Inputs=-+  InputSameDT=on  SaturateOnIntegerOverflow=on  OutDataTypeStr=Inherit: Same as first input
  Sum2 : Sum  Inputs=--  InputSameDT=on  SaturateOnIntegerOverflow=on  OutDataTypeStr=Inherit: Same as first input
  Sum3 : Sum  Inputs=--  InputSameDT=on  SaturateOnIntegerOverflow=on  OutDataTypeStr=Inherit: Same as first input
  Sum4 : Sum  Inputs=1  InputSameDT=on  SaturateOnIntegerOverflow=on  OutDataTypeStr=Inherit: Same as first input
  vq_s : Outport
  vd_s : Outport  Port=2
  vo_s : Outport  Port=3
  wires:
  Sum/1 -> Mux2/3, Sum2/1  "sin(wt-2pi/3)"
  Fcn1/1 -> vq_s/1  "Vq"
  Fcn3/1 -> Sum3/2, Product3/1, Product1/1, Mux2/2  "cos(wt)"
  K2/1 -> Product1/2, Product2/2
  Sum2/1 -> Mux2/5  "sin(wt+2pi/3)"
  Fcn/1 -> Product/1, Product2/1, Sum2/2, Mux2/1  "sin(wt)"
  Sum1/1 -> Mux2/4, Sum3/1  "cos(wt-2pi/3)"
  K1/1 -> Product/2, Product3/2
  Product1/1 -> Sum/2
  Product2/1 -> Sum1/2
  Mux2/1 -> Mux/2
  Product/1 -> Sum/1
  abc/1 -> Mux/1
  Sum4/1 -> Gain1/1
  Product3/1 -> Sum1/1
  Fcn2/1 -> vd_s/1  "Vd"
  Sum3/1 -> Mux2/6  "cos(wt+2pi/3)"
  theta_degree/1 -> Fcn3/1, Fcn/1
  Mux/1 -> Fcn2/1, Fcn1/1, Sum4/1
  Gain1/1 -> vo_s/1

== system PMSM_FOC_INVERTER_COMPARISON/PMSM2/Clarke_Park_Transformation/Park Transformation ==
  qs_s : Inport
  ds_s : Inport  Port=2
  cos theta_e : Inport  Port=3
  Sin theta_e : Inport  Port=4
  Add : Sum  Inputs=+-
  Add1 : Sum
  Product{,1..3} (4 alike) : Product  RndMeth=Zero
  qs_r : Outport
  ds_r : Outport  Port=2
  wires:
  cos theta_e/1 -> Product/2, Product2/2
  Sin theta_e/1 -> Product1/2, Product3/2
  Product1/1 -> Add/2
  ds_s/1 -> Product1/1, Product2/1
  Add1/1 -> ds_r/1
  Product/1 -> Add/1
  qs_s/1 -> Product/1, Product3/1
  Add/1 -> qs_r/1
  Product3/1 -> Add1/1
  Product2/1 -> Add1/2

== system PMSM_FOC_INVERTER_COMPARISON/PMSM2/Clarke_Park_Transformation/Subsystem ==
  theta_e : Inport
  Fcn : Fcn  Expr=sin(u)
  Fcn1 : Fcn  Expr=cos(u)
  cos : Outport
  sin : Outport  Port=2
  wires:
  theta_e/1 -> Fcn/1, Fcn1/1
  Fcn1/1 -> cos/1
  Fcn/1 -> sin/1

== system PMSM_FOC_INVERTER_COMPARISON/PMSM2/PMSM Dynamic Model/Electromagnetic Torque ==
  iq : Inport
  id : Inport  Port=2
  Add : Sum
  Gain : Gain  Gain=Ld-Lq
  Gain1 : Gain  Gain=(3/2)*P
  Gain2 : Gain  Gain=Lambda_m
  Product : Product
  Te : Outport
  wires:
  Add/1 -> Gain1/1
  Gain2/1 -> Add/2
  Product/1 -> Gain/1
  iq/1 -> Gain2/1, Product/1
  Gain/1 -> Add/1
  Gain1/1 -> Te/1
  id/1 -> Product/2

== system PMSM_FOC_INVERTER_COMPARISON/PMSM2/PMSM Dynamic Model/Subsystem ==
  Te : Inport
  TL : Inport  Port=2
  Gain : Gain  Gain=1/P
  Integrator : Integrator
  Mechanical_speed_calculations : Subsystem
  Omega_m : Outport
  Theta_m : Outport  Port=2
  Omega_e : Outport  Port=3
  Theta_e : Outport  Port=4
  wires:
  TL/1 -> Mechanical_speed_calculations/2(TL)
  Integrator/1 -> Theta_m/1
  Mechanical_speed_calculations/1(Omega_e) -> Gain/1, Omega_e/1
  Te/1 -> Mechanical_speed_calculations/1(Te)
  Mechanical_speed_calculations/2(Theta_e) -> Theta_e/1
  Gain/1 -> Integrator/1, Omega_m/1

== system PMSM_FOC_INVERTER_COMPARISON/PMSM2/PMSM Dynamic Model/iqd_calculations ==
  vq : Inport
  Omega_e : Inport  Port=2
  vd : Inport  Port=3
  id_calculations : Subsystem
  iq_calculations : Subsystem
  iq : Outport
  id : Outport  Port=2
  wires:
  vq/1 -> iq_calculations/1(vq)
  id_calculations/1(id) -> id/1, iq_calculations/3(id)
  Omega_e/1 -> iq_calculations/2(Omega_e), id_calculations/2(Omega_e)
  iq_calculations/1(iq) -> iq/1, id_calculations/3(iq)
  vd/1 -> id_calculations/1(vd)

== system PMSM_FOC_INVERTER_COMPARISON/PMSM1/PMSM Dynamic Model/Subsystem/Mechanical_speed_calculations ==
  Te : Inport
  TL : Inport  Port=2
  Add : Sum  Inputs=+--
  Gain : Gain  Gain=(P)*(1/J)
  Gain1 : Gain  Gain=B*(1/P)
  Integrator : Integrator
  Integrator1 : Integrator
  Omega_e : Outport
  Theta_e : Outport  Port=2
  wires:
  Integrator1/1 -> Theta_e/1
  TL/1 -> Add/2
  Gain1/1 -> Add/3
  Add/1 -> Gain/1
  Te/1 -> Add/1
  Gain/1 -> Integrator/1
  Integrator/1 -> Gain1/1, Omega_e/1, Integrator1/1

== system PMSM_FOC_INVERTER_COMPARISON/PMSM1/PMSM Dynamic Model/iqd_calculations/id_calculations ==
  vd : Inport
  Omega_e : Inport  Port=2
  iq : Inport  Port=3
  1/Ld : Gain  Gain=1/Ld
  Add : Sum  Inputs=++-
  Gain : Gain  Gain=Rs
  Integrator : Integrator
  Lq : Gain  Gain=Lq
  Product : Product
  id : Outport
  wires:
  iq/1 -> Product/2
  Product/1 -> Lq/1
  Omega_e/1 -> Product/1
  Add/1 -> 1/Ld/1
  Gain/1 -> Add/3
  Integrator/1 -> Gain/1, id/1
  vd/1 -> Add/1
  Lq/1 -> Add/2
  1/Ld/1 -> Integrator/1

== system PMSM_FOC_INVERTER_COMPARISON/PMSM1/PMSM Dynamic Model/iqd_calculations/iq_calculations ==
  vq : Inport
  Omega_e : Inport  Port=2
  id : Inport  Port=3
  1/Lq : Gain  Gain=1/Lq
  Add : Sum  Inputs=+---
  Gain : Gain  Gain=Rs
  Gain1 : Gain  Gain=Lambda_m
  Integrator : Integrator
  Ld : Gain  Gain=Ld
  Product : Product
  iq : Outport
  wires:
  Gain1/1 -> Add/2
  id/1 -> Product/2
  Omega_e/1 -> Product/1, Gain1/1
  Ld/1 -> Add/3
  Gain/1 -> Add/4
  vq/1 -> Add/1
  Product/1 -> Ld/1
  1/Lq/1 -> Integrator/1
  Add/1 -> 1/Lq/1
  Integrator/1 -> Gain/1, iq/1

== system PMSM_FOC_INVERTER_COMPARISON/PMSM2/PMSM Dynamic Model/Subsystem/Mechanical_speed_calculations ==
  Te : Inport
  TL : Inport  Port=2
  Add : Sum  Inputs=+--
  Gain : Gain  Gain=(P)*(1/J)
  Gain1 : Gain  Gain=B*(1/P)
  Integrator : Integrator
  Integrator1 : Integrator
  Omega_e : Outport
  Theta_e : Outport  Port=2
  wires:
  Integrator/1 -> Integrator1/1, Omega_e/1, Gain1/1
  Gain/1 -> Integrator/1
  Te/1 -> Add/1
  Add/1 -> Gain/1
  Gain1/1 -> Add/3
  TL/1 -> Add/2
  Integrator1/1 -> Theta_e/1

== system PMSM_FOC_INVERTER_COMPARISON/PMSM2/PMSM Dynamic Model/iqd_calculations/id_calculations ==
  vd : Inport
  Omega_e : Inport  Port=2
  iq : Inport  Port=3
  1/Ld : Gain  Gain=1/Ld
  Add : Sum  Inputs=++-
  Gain : Gain  Gain=Rs
  Integrator : Integrator
  Lq : Gain  Gain=Lq
  Product : Product
  id : Outport
  wires:
  1/Ld/1 -> Integrator/1
  Lq/1 -> Add/2
  vd/1 -> Add/1
  Integrator/1 -> id/1, Gain/1
  Gain/1 -> Add/3
  Add/1 -> 1/Ld/1
  Omega_e/1 -> Product/1
  Product/1 -> Lq/1
  iq/1 -> Product/2

== system PMSM_FOC_INVERTER_COMPARISON/PMSM2/PMSM Dynamic Model/iqd_calculations/iq_calculations ==
  vq : Inport
  Omega_e : Inport  Port=2
  id : Inport  Port=3
  1/Lq : Gain  Gain=1/Lq
  Add : Sum  Inputs=+---
  Gain : Gain  Gain=Rs
  Gain1 : Gain  Gain=Lambda_m
  Integrator : Integrator
  Ld : Gain  Gain=Ld
  Product : Product
  iq : Outport
  wires:
  Integrator/1 -> iq/1, Gain/1
  Add/1 -> 1/Lq/1
  1/Lq/1 -> Integrator/1
  Product/1 -> Ld/1
  vq/1 -> Add/1
  Gain/1 -> Add/4
  Ld/1 -> Add/3
  Omega_e/1 -> Gain1/1, Product/1
  id/1 -> Product/2
  Gain1/1 -> Add/2
